simulink subsystem "BicycleWithForceInput"  (R2022b)
settings: Solver=VariableStepAuto  StartTime=0.0  StopTime=10.0  RelTol=1e-3
undefined symbols (not defined in the file): egoActorID, lr, m, max_ac, max_dc, tau, tau2, Ts
libraries: autolibshared x1
settings Model: Creator=The MathWorks, Inc.  LastModifiedBy=yunuo
settings SolverCC: MaxZcPerStep=1
settings DebuggingCC: UnconnectedInputMsg=warning  UnconnectedOutputMsg=warning  UnconnectedLineMsg=warning
settings ModelReferenceCC: EnableRefExpFcnMdlSchedulingChecks=on
settings RTWCC: DLArmComputeVersion=19.05

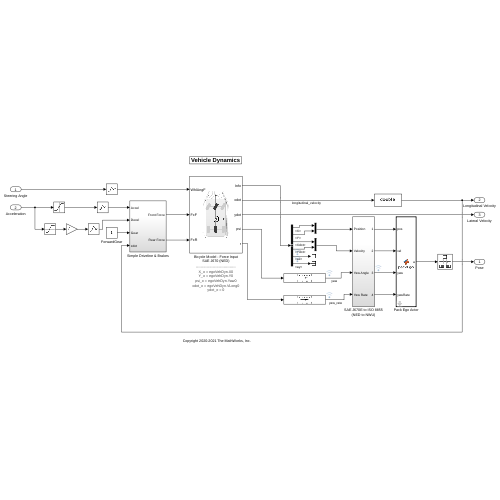
[thumbnail: Simulink's stored preview of the top-level diagram]
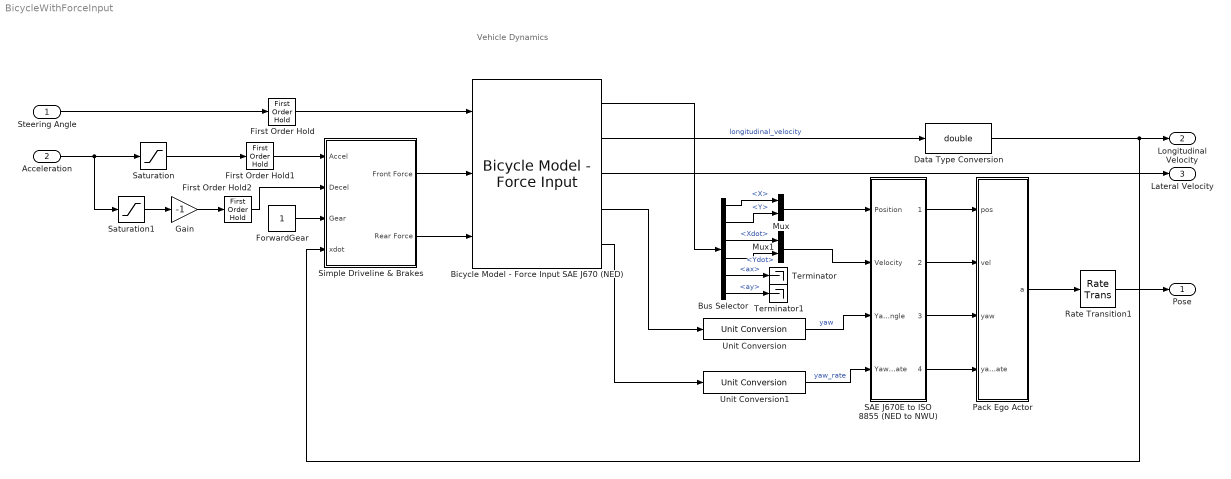
== system BicycleWithForceInput ==
  note: Vehicle Dynamics
  Steering Angle : Inport  Unit=rad
  Acceleration : Inport  Port=2  Unit=m/s^2
  Bicycle Model - Force Input SAE J670 (NED) : autolibshared/Bicycle Model - Force Input  trackMode=Single (bicycle)  inputMode=External longitudinal forces  frontSteerMode=on  rearSteerMode=off  windMode=off  muMode=off  extFMode=off  extMMode=off  aMode=3  NF=2  NR=2  m=m  a=lf  b=lr  h=0.35  X_o=egoVehDyn.X0  xdot_o=egoVehDyn.VLong0  CalphaMode=off  sigmaMode=on  w=[1.4,1.4]  Cy_f=Cf  Cy_r=Cr  sigma_f=.1  sigma_r=.1  alpha_f_brk=[-.1 .1]  Cy_f_data=[-9e3 9e3]  alpha_r_brk=[-.1 .1]  Cy_r_data=[-9e3 9e3]  Y_o=egoVehDyn.Y0  ydot_o=0  Izz=Iz  psi_o=egoVehDyn.Yaw0  r_o=0  Af=0  Cd=.3  Cl=.1  Cpm=.1  beta_w=[0:0.01:0.3]  Cs=[0:0.03:0.9]  Cym=[0:0.01:0.3]  Pabs=101325  Tair=273  g=9.81  mu=1  xdot_tol=.01  Fznom=5000  Fxtire_sat=1e6  Fytire_sat=1e6  longOff=0  latOff=0  vertOff=0
      settings: AttributesFormatString=|
      | ---------------------------------
      | X_o = %<X_o>
      | Y_o = %<Y_o>
      | psi_o = %<psi_o>
      | xdot_o = %<xdot_o>
      | ydot_o = %<ydot_o>
  Bus Selector : BusSelector  OutputSignals=InertFrm.RearAxl.Disp.X,InertFrm.RearAxl.Disp.Y,InertFrm.RearAxl.Vel.Xdot,InertFrm.RearAxl.Vel.Ydot,BdyFrm.Cg.Acc.ax,BdyFrm.Cg.Acc.ay
  Data Type Conversion : DataTypeConversion  OutDataTypeStr=double  SaturateOnIntegerOverflow=off  RndMeth=Floor
  First Order Hold : FirstOrderHold  ErrorTolerance=inf
  First Order Hold1 : FirstOrderHold  ErrorTolerance=inf
  First Order Hold2 : FirstOrderHold  ErrorTolerance=inf
  ForwardGear : Constant  SampleTime=Ts
  Gain : Gain  Gain=-1
  Mux : Mux  Inputs=2
  Mux1 : Mux  Inputs=2
  Pack Ego Actor : MATLAB Function  TreatAsAtomicUnit=on  mask{egoActorID=egoActorID}
      mask prompts: egoActorID "Ego Actor ID"
  Rate Transition1 : RateTransition  OutPortSampleTime=Ts
  SAE J670E to ISO 8855 (NED to NWU) : Subsystem
  Saturation : Saturate  UpperLimit=max_ac  LowerLimit=0
  Saturation1 : Saturate  UpperLimit=0  LowerLimit=max_dc
  Simple Driveline & Brakes : Subsystem
  Terminator : Terminator
  Terminator1 : Terminator
  Unit Conversion : UnitConversion  OutputType=Inherit: Inherit via back propagation
  Unit Conversion1 : UnitConversion  OutputType=Inherit: Inherit via back propagation
  Pose : Outport  VectorParamsAs1DForOutWhenUnconnected=off
  Longitudinal Velocity : Outport  Port=2  Unit=m/s  VectorParamsAs1DForOutWhenUnconnected=off
  Lateral Velocity : Outport  Port=3  Unit=m/s  VectorParamsAs1DForOutWhenUnconnected=off
  wires:
  Bicycle Model - Force Input SAE J670 (NED)/2 -> Data Type Conversion/1  "longitudinal_velocity"
  Data Type Conversion/1 -> Longitudinal Velocity/1, Simple Driveline & Brakes/4(xdot)
  Bus Selector/3 -> Mux1/1  "<Xdot>"
  Bicycle Model - Force Input SAE J670 (NED)/1 -> Bus Selector/1
  SAE J670E to ISO 8855 (NED to NWU)/4(4) -> Pack Ego Actor/4(yawRate)
  Bicycle Model - Force Input SAE J670 (NED)/5 -> Unit Conversion1/1
  SAE J670E to ISO 8855 (NED to NWU)/3(3) -> Pack Ego Actor/3(yaw)
  Bus Selector/1 -> Mux/1  "<X>"
  Mux/1 -> SAE J670E to ISO 8855 (NED to NWU)/1(Position)
  Pack Ego Actor/1(a) -> Rate Transition1/1
  Bus Selector/2 -> Mux/2  "<Y>"
  Bicycle Model - Force Input SAE J670 (NED)/4 -> Unit Conversion/1
  Mux1/1 -> SAE J670E to ISO 8855 (NED to NWU)/2(Velocity)
  SAE J670E to ISO 8855 (NED to NWU)/2(2) -> Pack Ego Actor/2(vel)
  Unit Conversion1/1 -> SAE J670E to ISO 8855 (NED to NWU)/4(Yaw Rate)  "yaw_rate"
  Bus Selector/4 -> Mux1/2  "<Ydot>"
  Unit Conversion/1 -> SAE J670E to ISO 8855 (NED to NWU)/3(Yaw Angle)  "yaw"
  SAE J670E to ISO 8855 (NED to NWU)/1(1) -> Pack Ego Actor/1(pos)
  Rate Transition1/1 -> Pose/1
  Bicycle Model - Force Input SAE J670 (NED)/3 -> Lateral Velocity/1
  ForwardGear/1 -> Simple Driveline & Brakes/3(Gear)
  Simple Driveline & Brakes/1(Front Force) -> Bicycle Model - Force Input SAE J670 (NED)/2
  Simple Driveline & Brakes/2(Rear Force) -> Bicycle Model - Force Input SAE J670 (NED)/3
  Steering Angle/1 -> First Order Hold/1
  Saturation/1 -> First Order Hold1/1
  Gain/1 -> First Order Hold2/1
  Acceleration/1 -> Saturation/1, Saturation1/1
  Saturation1/1 -> Gain/1
  First Order Hold1/1 -> Simple Driveline & Brakes/1(Accel)
  First Order Hold/1 -> Bicycle Model - Force Input SAE J670 (NED)/1
  First Order Hold2/1 -> Simple Driveline & Brakes/2(Decel)
  Bus Selector/5 -> Terminator/1  "<ax>"
  Bus Selector/6 -> Terminator1/1  "<ay>"

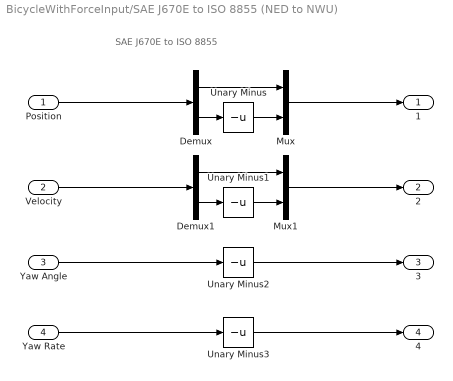
== system BicycleWithForceInput/SAE J670E to ISO 8855 (NED to NWU) ==
  note: SAE J670E to ISO 8855
  Position : Inport  Unit=m
  Velocity : Inport  Port=2  Unit=m/s
  Yaw Angle : Inport  Port=3  Unit=deg
  Yaw Rate : Inport  Port=4  Unit=deg/s
  Demux : Demux  Outputs=2
  Demux1 : Demux  Outputs=2
  Mux : Mux  Inputs=2
  Mux1 : Mux  Inputs=2
  Unary Minus{,1..3} (4 alike) : UnaryMinus
  1 : Outport  VectorParamsAs1DForOutWhenUnconnected=off
  2 : Outport  Port=2  VectorParamsAs1DForOutWhenUnconnected=off
  3 : Outport  Port=3  VectorParamsAs1DForOutWhenUnconnected=off
  4 : Outport  Port=4  VectorParamsAs1DForOutWhenUnconnected=off
  wires:
  Unary Minus3/1 -> 4/1
  Unary Minus2/1 -> 3/1
  Velocity/1 -> Demux1/1
  Position/1 -> Demux/1
  Mux/1 -> 1/1
  Mux1/1 -> 2/1
  Demux1/1 -> Mux1/1
  Demux1/2 -> Unary Minus1/1
  Unary Minus1/1 -> Mux1/2
  Unary Minus/1 -> Mux/2
  Demux/2 -> Unary Minus/1
  Demux/1 -> Mux/1
  Yaw Angle/1 -> Unary Minus2/1
  Yaw Rate/1 -> Unary Minus3/1

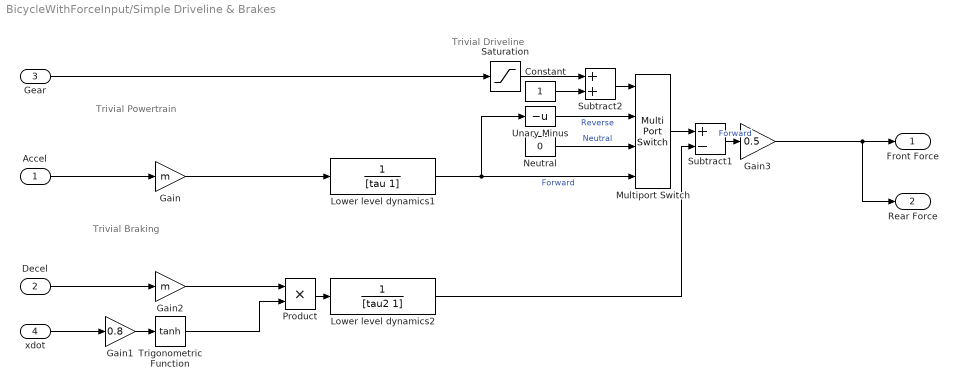
== system BicycleWithForceInput/Simple Driveline & Brakes ==
  note: Trivial Braking
  note: Trivial Powertrain
  note: Trivial Driveline
  Accel : Inport
  Decel : Inport  Port=2
  Gear : Inport  Port=3
  xdot : Inport  Port=4
  Constant : Constant
  Gain : Gain  Gain=m
  Gain1 : Gain  Gain=0.8
  Gain2 : Gain  Gain=m
  Gain3 : Gain  Gain=0.5
  Lower level dynamics1 : TransferFcn  Denominator=[tau 1]
  Lower level dynamics2 : TransferFcn  Denominator=[tau2 1]
  Multiport Switch : MultiPortSwitch  DataPortOrder=Zero-based contiguous  zeroidx=on  SaturateOnIntegerOverflow=off  InputSameDT=off
  Neutral : Constant  Value=0
  Product : Product
  Saturation : Saturate  UpperLimit=1  LowerLimit=-1  ZeroCross=off
  Subtract1 : Sum  Inputs=+-
  Subtract2 : Sum
  Trigonometric Function : Trigonometry  Operator=tanh
  Unary Minus : UnaryMinus
  Front Force : Outport  VectorParamsAs1DForOutWhenUnconnected=off
  Rear Force : Outport  Port=2  VectorParamsAs1DForOutWhenUnconnected=off
  wires:
  Gain3/1 -> Rear Force/1, Front Force/1
  Unary Minus/1 -> Multiport Switch/2  "Reverse"
  Subtract1/1 -> Gain3/1  "Forward"
  Saturation/1 -> Subtract2/1
  Lower level dynamics1/1 -> Multiport Switch/4, Unary Minus/1  "Forward"
  Neutral/1 -> Multiport Switch/3  "Neutral"
  Subtract2/1 -> Multiport Switch/1
  Constant/1 -> Subtract2/2
  Gear/1 -> Saturation/1
  Product/1 -> Lower level dynamics2/1
  Lower level dynamics2/1 -> Subtract1/2
  Gain2/1 -> Product/1
  Gain/1 -> Lower level dynamics1/1
  Gain1/1 -> Trigonometric Function/1
  Trigonometric Function/1 -> Product/2
  Decel/1 -> Gain2/1
  xdot/1 -> Gain1/1
  Accel/1 -> Gain/1
  Multiport Switch/1 -> Subtract1/1

== matlab function BicycleWithForceInput/Pack Ego Actor ==
  data: pos input; a output Bus: BusVehiclePose size=1; vel input; yaw input; yawRate input; egoActorID parameter
function a = packEgo(pos,vel,yaw,yawRate, egoActorID)
% Pack ego information into a single ego actor bus
%
% Important note:
% Output is a bus of type BusVehiclePose. This bus must match the bus 
% elements expected by Scenario Reader. You can view the 
% bus association using 'Edit Data' in the menu above.

a = struct(...
    'ActorID', egoActorID,...
    'Position', [pos(1) pos(2) 0], ...
    'Velocity', [vel(1) vel(2) 0], ...
    'Roll', 0, ...
    'Pitch', 0, ...
    'Yaw', yaw, ...
    'AngularVelocity', [0 0 yawRate]);
